simulink model "Test_Multiplexer_Demultiplexer"  (Simulink 8.1)
settings: Solver=ode45  StartTime=0.0  StopTime=10.0  RelTol=1e-3
libraries: Computer_Library x12, commutil2 x5
settings Model: Creator=N  LastModifiedBy=uzivatel
settings DataIOCC: LimitDataPoints=off  SignalLoggingSaveFormat=Dataset
settings OptimizationCC: ExpressionDepthLimit=128
settings DebuggingCC: UnderspecifiedInitializationDetection=Simplified  MergeDetectMultiDrivingBlocksExec=error  SolverPrmCheckMsg=none  FcnCallInpInsideContextMsg=EnableAllAsError  FrameProcessingCompatibilityMsg=error  StateNameClashWarn=none
settings HardwareCC: ProdBitPerPointer=64  ProdLargestAtomicFloat=Float  ProdIntDivRoundTo=Zero  ProdEndianess=LittleEndian  ProdHWDeviceType=Intel->x86-64 (Windows64)
settings ModelReferenceCC: PropagateSignalLabelsOutOfModel=on
settings GRTTargetCC: CodeReplacementLibrary=None  CombineOutputUpdateFcns=on  CPPClassGenCompliant=on  GRTInterface=off

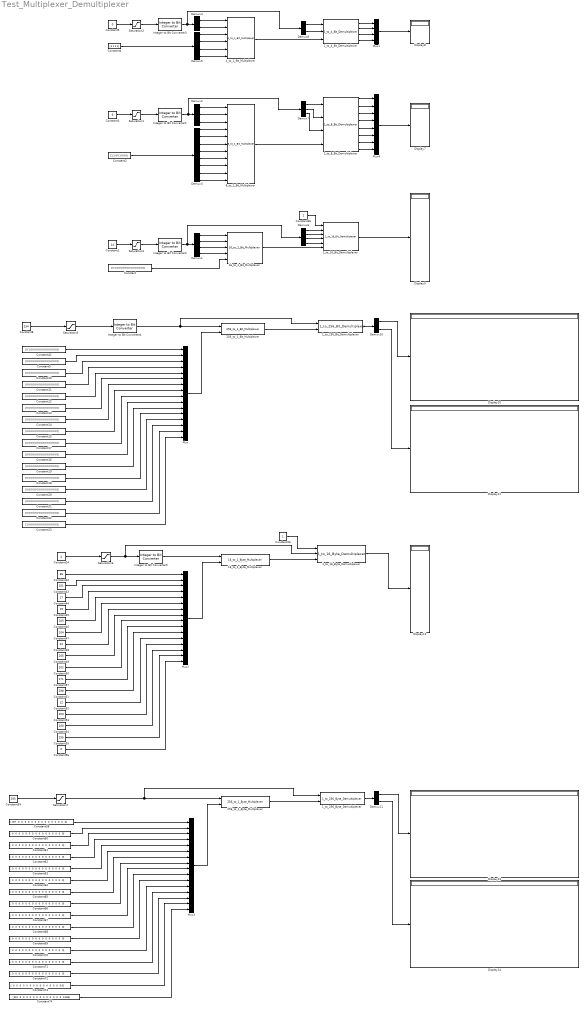
== system Test_Multiplexer_Demultiplexer ==
  16_to_1_Bit_Multiplexer : Computer_Library/Multiplexers/16_to_1_Bit_Multiplexer
  16_to_1_Byte_Multiplexer : Computer_Library/Multiplexers/16_to_1_Byte_Multiplexer
  1_to_16_Bit_Demultiplexer : Computer_Library/Demultiplexers/1_to_16_Bit_Demultiplexer
  1_to_16_Byte_Demultiplexer : Computer_Library/Demultiplexers/1_to_16_Byte_Demultiplexer
  1_to_256_Bit_Demultiplexer : Computer_Library/Demultiplexers/1_to_256_Bit_Demultiplexer
  1_to_256_Byte_Demultiplexer : Computer_Library/Demultiplexers/1_to_256_Byte_Demultiplexer
  1_to_4_Bit_Demultiplexer : Computer_Library/Demultiplexers/1_to_4_Bit_Demultiplexer
  1_to_8_Bit_Demultiplexer : Computer_Library/Demultiplexers/1_to_8_Bit_Demultiplexer
  256_to_1_Bit_Multiplexer : Computer_Library/Multiplexers/256_to_1_Bit_Multiplexer
  256_to_1_Byte_Multiplexer : Computer_Library/Multiplexers/256_to_1_Byte_Multiplexer
  4_to_1_Bit_Multiplexer : Computer_Library/Multiplexers/4_to_1_Bit_Multiplexer
  8_to_1_Bit_Multiplexer : Computer_Library/Multiplexers/8_to_1_Bit_Multiplexer
  Constant : Constant  Value=[0 1 0 0 0 0 0 0 0 0 0 0 0 0 0 0]
  Constant1 : Constant  Value=14
  Constant{9..22} (14 alike) : Constant  Value=[0 0 0 0 0 0 0 0 0 0 0 0 0 0 0 0]  OutDataTypeStr=uint8
  Constant2 : Constant  Value=[1 1 0 0 1 0 0 0]
  Constant23 : Constant  Value=[1 0 0 0 0 0 0 0 0 0 0 0 0 0 0 0]  OutDataTypeStr=uint8
  Constant24 : Constant  Value=4  OutDataTypeStr=uint8
  Constant26 : Constant
  Constant3 : Constant  Value=6
  Constant36 : Constant
  Constant4 : Constant  Value=[1 1 1 1]
  Constant41 : Constant  Value=[0 1 0 0 0 0 0 0 0 0 0 0 0 0 0 0]  OutDataTypeStr=uint8
  Constant42 : Constant  Value=66  OutDataTypeStr=uint8
  Constant43 : Constant  Value=151  OutDataTypeStr=uint8
  Constant44 : Constant  Value=17  OutDataTypeStr=uint8
  Constant45 : Constant  Value=19  OutDataTypeStr=uint8
  Constant46 : Constant  Value=105  OutDataTypeStr=uint8
  Constant47 : Constant  Value=104  OutDataTypeStr=uint8
  Constant48 : Constant  Value=22  OutDataTypeStr=uint8
  Constant49 : Constant  Value=205  OutDataTypeStr=uint8
  Constant5 : Constant  Value=0
  Constant50 : Constant  Value=202  OutDataTypeStr=uint8
  Constant51 : Constant  Value=198  OutDataTypeStr=uint8
  Constant52 : Constant  Value=12  OutDataTypeStr=uint8
  Constant53 : Constant  Value=200  OutDataTypeStr=uint8
  Constant54 : Constant  Value=100  OutDataTypeStr=uint8
  Constant55 : Constant  Value=255  OutDataTypeStr=uint8
  Constant56 : Constant  Value=0  OutDataTypeStr=uint8
  Constant57 : Constant  Value=171  OutDataTypeStr=uint8
  Constant58 : Constant  Value="[  207   0   0   0   0   0   0   0   0   0   0   0   0   0   0   0]"  OutDataTypeStr=uint8
  Constant59 : Constant  Value=255  OutDataTypeStr=uint8
  Constant{60..72} (13 alike) : Constant  Value="[  0   0   0   0   0   0   0   0   0   0   0   0   0   0   0   0]"  OutDataTypeStr=uint8
  Constant73 : Constant  Value="[  0   0   0   0   0   0   0   0   0   0   0   0   0   0   0 0]"  OutDataTypeStr=uint8
  Constant74 : Constant  Value="[113   0   0   0   0   0   0   0   0   0   0   0   0   0   0 255]"  OutDataTypeStr=uint8
  Constant8 : Constant  Value=254  OutDataTypeStr=uint8
  Demux1 : Demux
  Demux{4,8,10..11} (4 alike) : Demux  Outputs=2
  Demux2 : Demux  Outputs=3
  Demux3 : Demux  Outputs=8
  Demux5 : Demux
  Demux6 : Demux
  Demux7 : Demux  Outputs=3
  Display{7..14} (8 alike) : Display
  Integer to Bit Converter1 : commutil2/Integer to Bit Converter  nbits=3  signedInputValues=Unsigned  bitOrder=MSB first  outDtype=uint8
  Integer to Bit Converter2 : commutil2/Integer to Bit Converter  nbits=4  signedInputValues=Unsigned  bitOrder=MSB first  outDtype=int8
  Integer to Bit Converter3 : commutil2/Integer to Bit Converter  nbits=2  signedInputValues=Unsigned  bitOrder=MSB first  outDtype=boolean
  Integer to Bit Converter4 : commutil2/Integer to Bit Converter  nbits=8  signedInputValues=Unsigned  bitOrder=MSB first  outDtype=boolean
  Integer to Bit Converter5 : commutil2/Integer to Bit Converter  nbits=4  signedInputValues=Unsigned  bitOrder=MSB first  outDtype=boolean
  Mux : Mux  Inputs=16
  Mux1 : Mux
  Mux2 : Mux  Inputs=16
  Mux3 : Mux  Inputs=16
  Mux4 : Mux  Inputs=8
  Saturation1 : Saturate  UpperLimit=7  LowerLimit=0
  Saturation2 : Saturate  UpperLimit=3  LowerLimit=0
  Saturation3 : Saturate  UpperLimit=15  LowerLimit=0
  Saturation5 : Saturate  UpperLimit=255  LowerLimit=0
  Saturation6 : Saturate  UpperLimit=15  LowerLimit=0
  Saturation7 : Saturate  UpperLimit=255  LowerLimit=0
  wires:
  Constant/1 -> 16_to_1_Bit_Multiplexer/5
  Demux1/1 -> 16_to_1_Bit_Multiplexer/1
  Demux1/2 -> 16_to_1_Bit_Multiplexer/2
  Demux1/3 -> 16_to_1_Bit_Multiplexer/3
  Demux1/4 -> 16_to_1_Bit_Multiplexer/4
  Constant1/1 -> Saturation3/1
  Saturation3/1 -> Integer to Bit Converter2/1
  Constant2/1 -> Demux3/1
  Integer to Bit Converter1/1 -> Demux7/1, Demux2/1
  Constant3/1 -> Saturation1/1
  Saturation1/1 -> Integer to Bit Converter1/1
  Demux3/1 -> 8_to_1_Bit_Multiplexer/4
  Demux3/2 -> 8_to_1_Bit_Multiplexer/5
  Demux3/3 -> 8_to_1_Bit_Multiplexer/6
  Demux3/4 -> 8_to_1_Bit_Multiplexer/7
  Demux3/5 -> 8_to_1_Bit_Multiplexer/8
  Demux3/6 -> 8_to_1_Bit_Multiplexer/9
  Demux3/7 -> 8_to_1_Bit_Multiplexer/10
  Demux3/8 -> 8_to_1_Bit_Multiplexer/11
  Constant4/1 -> Demux5/1
  Integer to Bit Converter3/1 -> Demux8/1, Demux4/1
  Constant5/1 -> Saturation2/1
  Saturation2/1 -> Integer to Bit Converter3/1
  Demux5/1 -> 4_to_1_Bit_Multiplexer/3
  Demux5/2 -> 4_to_1_Bit_Multiplexer/4
  Demux5/3 -> 4_to_1_Bit_Multiplexer/5
  Demux5/4 -> 4_to_1_Bit_Multiplexer/6
  Constant41/1 -> Mux/1
  Constant9/1 -> Mux/2
  Constant10/1 -> Mux/3
  Constant11/1 -> Mux/4
  Constant12/1 -> Mux/5
  Constant23/1 -> Mux/16
  Constant22/1 -> Mux/15
  Constant21/1 -> Mux/14
  Constant20/1 -> Mux/13
  Constant18/1 -> Mux/12
  Constant19/1 -> Mux/11
  Constant16/1 -> Mux/10
  Constant17/1 -> Mux/9
  Constant15/1 -> Mux/8
  Constant14/1 -> Mux/7
  Constant13/1 -> Mux/6
  Mux/1 -> 256_to_1_Bit_Multiplexer/2
  Saturation5/1 -> Integer to Bit Converter4/1
  Constant8/1 -> Saturation5/1
  Constant24/1 -> Saturation6/1
  Integer to Bit Converter5/1 -> 16_to_1_Byte_Multiplexer/1
  Constant42/1 -> Mux2/1
  Constant43/1 -> Mux2/2
  Constant44/1 -> Mux2/3
  Constant45/1 -> Mux2/4
  Constant46/1 -> Mux2/5
  Constant56/1 -> Mux2/16
  Constant55/1 -> Mux2/15
  Constant54/1 -> Mux2/14
  Constant53/1 -> Mux2/13
  Constant52/1 -> Mux2/12
  Constant51/1 -> Mux2/11
  Constant57/1 -> Mux2/10
  Constant50/1 -> Mux2/9
  Constant49/1 -> Mux2/8
  Constant48/1 -> Mux2/7
  Constant47/1 -> Mux2/6
  Mux2/1 -> 16_to_1_Byte_Multiplexer/2
  16_to_1_Byte_Multiplexer/1 -> 1_to_16_Byte_Demultiplexer/3
  Constant59/1 -> Saturation7/1
  Constant58/1 -> Mux3/1
  Constant60/1 -> Mux3/2
  Constant61/1 -> Mux3/3
  Constant62/1 -> Mux3/4
  Constant63/1 -> Mux3/5
  Constant74/1 -> Mux3/16
  Constant73/1 -> Mux3/15
  Constant72/1 -> Mux3/14
  Constant71/1 -> Mux3/13
  Constant70/1 -> Mux3/12
  Constant69/1 -> Mux3/11
  Constant68/1 -> Mux3/10
  Constant67/1 -> Mux3/9
  Constant66/1 -> Mux3/8
  Constant65/1 -> Mux3/7
  Constant64/1 -> Mux3/6
  Mux3/1 -> 256_to_1_Byte_Multiplexer/2
  Demux6/1 -> 1_to_16_Bit_Demultiplexer/2
  Demux6/2 -> 1_to_16_Bit_Demultiplexer/3
  Demux6/3 -> 1_to_16_Bit_Demultiplexer/4
  Demux6/4 -> 1_to_16_Bit_Demultiplexer/5
  Integer to Bit Converter2/1 -> Demux6/1, Demux1/1
  16_to_1_Bit_Multiplexer/1 -> 1_to_16_Bit_Demultiplexer/6
  1_to_16_Bit_Demultiplexer/1 -> Display9/1
  Demux2/1 -> 8_to_1_Bit_Multiplexer/1
  Demux2/2 -> 8_to_1_Bit_Multiplexer/2
  Demux2/3 -> 8_to_1_Bit_Multiplexer/3
  8_to_1_Bit_Multiplexer/1 -> 1_to_8_Bit_Demultiplexer/4
  Demux4/1 -> 4_to_1_Bit_Multiplexer/1
  Demux4/2 -> 4_to_1_Bit_Multiplexer/2
  4_to_1_Bit_Multiplexer/1 -> 1_to_4_Bit_Demultiplexer/3
  1_to_4_Bit_Demultiplexer/1 -> Mux1/1
  1_to_4_Bit_Demultiplexer/2 -> Mux1/2
  1_to_4_Bit_Demultiplexer/3 -> Mux1/3
  1_to_4_Bit_Demultiplexer/4 -> Mux1/4
  1_to_8_Bit_Demultiplexer/1 -> Mux4/1
  1_to_8_Bit_Demultiplexer/8 -> Mux4/8
  1_to_8_Bit_Demultiplexer/2 -> Mux4/2
  1_to_8_Bit_Demultiplexer/3 -> Mux4/3
  1_to_8_Bit_Demultiplexer/4 -> Mux4/4
  1_to_8_Bit_Demultiplexer/5 -> Mux4/5
  1_to_8_Bit_Demultiplexer/6 -> Mux4/6
  1_to_8_Bit_Demultiplexer/7 -> Mux4/7
  Mux4/1 -> Display7/1
  Mux1/1 -> Display8/1
  Constant36/1 -> 1_to_16_Bit_Demultiplexer/1
  256_to_1_Bit_Multiplexer/1 -> 1_to_256_Bit_Demultiplexer/2
  Integer to Bit Converter4/1 -> 1_to_256_Bit_Demultiplexer/1, 256_to_1_Bit_Multiplexer/1
  1_to_256_Bit_Demultiplexer/1 -> Demux10/1
  Demux10/1 -> Display10/1
  Demux10/2 -> Display11/1
  Constant26/1 -> 1_to_16_Byte_Demultiplexer/1
  Saturation6/1 -> 1_to_16_Byte_Demultiplexer/2, Integer to Bit Converter5/1
  1_to_16_Byte_Demultiplexer/1 -> Display12/1
  1_to_256_Byte_Demultiplexer/1 -> Demux11/1
  Demux11/1 -> Display13/1
  Demux11/2 -> Display14/1
  Saturation7/1 -> 1_to_256_Byte_Demultiplexer/1, 256_to_1_Byte_Multiplexer/1
  256_to_1_Byte_Multiplexer/1 -> 1_to_256_Byte_Demultiplexer/2
  Demux7/1 -> 1_to_8_Bit_Demultiplexer/1
  Demux7/2 -> 1_to_8_Bit_Demultiplexer/2
  Demux7/3 -> 1_to_8_Bit_Demultiplexer/3
  Demux8/2 -> 1_to_4_Bit_Demultiplexer/2
  Demux8/1 -> 1_to_4_Bit_Demultiplexer/1
